simulink model "DFF"  (R2015b)
settings: Solver=ode45  StartTime=0.0  StopTime=100.0  RelTol=1e-3
libraries: simulink_extras x1, commutil2 x1
settings Model: Creator=narayan  LastModifiedBy=RamPrasadh
settings DataIOCC: SaveFormat=Array
settings DebuggingCC: SolverPrmCheckMsg=warning
settings HardwareCC: ProdBitPerPointer=32  ProdLargestAtomicFloat=None  ProdIntDivRoundTo=Undefined  ProdEndianess=Unspecified  ProdWordSize=32  ProdHWDeviceType=32-bit Generic
settings GRTTargetCC: GeneratePreprocessorConditionals=Disable all
settings ConfigComp: CovModelRefEnable=Off  CovSFcnEnable=off

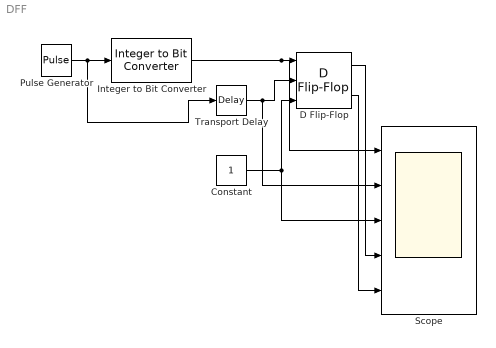
== system DFF ==
  Constant : Constant  OutDataTypeStr=boolean
  D Flip-Flop : simulink_extras/Flip Flops/D Flip-Flop
  Integer to Bit Converter : commutil2/Integer to Bit Converter  nbits=1  signedInputValues=Unsigned  bitOrder=MSB first  outDtype=boolean
  Pulse Generator : DiscretePulseGenerator  PulseType=Time based  Period=10  PulseWidth=7  PhaseDelay=2
  Scope : Scope  NumInputPorts=5
  Transport Delay : TransportDelay  DelayTime=2
  wires:
  Pulse Generator/1 -> Transport Delay/1, Integer to Bit Converter/1
  Integer to Bit Converter/1 -> Scope/1, D Flip-Flop/1
  Transport Delay/1 -> Scope/2, D Flip-Flop/2
  Constant/1 -> D Flip-Flop/3, Scope/3
  D Flip-Flop/1 -> Scope/4
  D Flip-Flop/2 -> Scope/5
